simulink model "jacobian"  (R2024b)
settings: Solver=ode1  StartTime=0.0  StopTime=inf  FixedStep=dt  MaxStep=1/30  RelTol=1e-3
undefined symbols (not defined in the file or in its folder): alpha, f, J_inv, y0
libraries: instrumentlib x2, simulink x1
settings Model: Creator=root  LastModifiedBy=aalessan

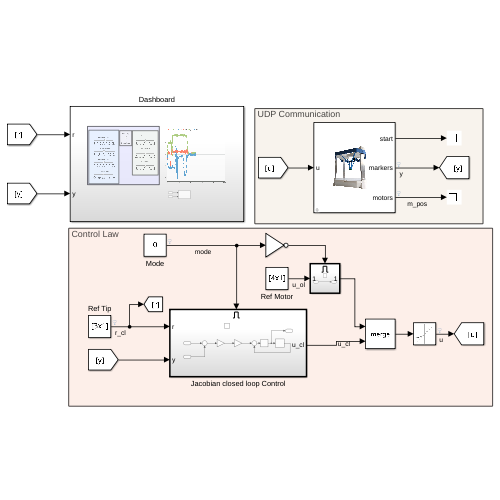
[thumbnail: Simulink's stored preview of the top-level diagram]
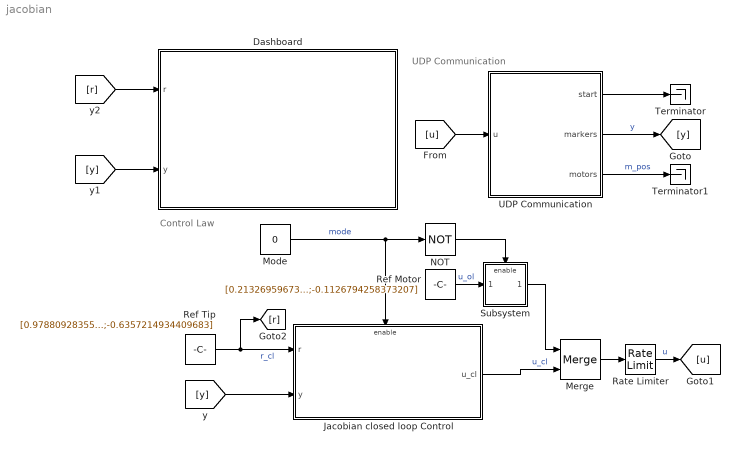
== system jacobian ==
  note: Control Law
  note: UDP Communication
  Dashboard : Subsystem
  Jacobian closed loop Control : Subsystem
  Merge : Merge  InitialOutput=zeros(4,1)
  Mode : Constant  Value=0
  NOT : Logic  Operator=NOT  IconShape=distinctive  AllPortsSameDT=off  OutDataTypeStr=boolean
  Rate Limiter : RateLimiter  RisingSlewLimit=7.906  FallingSlewLimit=-7.906  SampleTimeMode=inherited
  Ref Motor : Constant  Value=[0.213269596737653;-0.0957361805523107;-0.041409661167638;-0.1126794258373207]
  Ref Tip : Constant  Value=[0.9788092835519606;1.947527749747735;-0.6357214934409683]
  Subsystem : Subsystem
  Terminator : Terminator
  Terminator1 : Terminator
  UDP Communication : Subsystem  mask{nb_markers=1, markers_init=y0}
      mask prompts: nb_markers "Nb Markers"; markers_init "Initial Markers Position"
      mask Display: image('emio.png', [0,0,10,0,50,50]);
  wires:
  Merge/1 -> Rate Limiter/1
  Jacobian closed loop Control/1(u_cl) -> Merge/2  "u_cl"
  [u] -> UDP Communication/1(u)
  [y] -> Jacobian closed loop Control/2(y)
  Ref Tip/1 -> [r], Jacobian closed loop Control/1(r)  "r_cl"
  NOT/1 -> Subsystem/Enable
  Ref Motor/1 -> Subsystem/1(In1)  "u_ol"
  Mode/1 -> NOT/1, Jacobian closed loop Control/Enable  "mode"
  Subsystem/1(Out1) -> Merge/1
  Rate Limiter/1 -> [u]  "u"
  UDP Communication/3(motors) -> Terminator1/1  "m_pos"
  UDP Communication/1(start) -> Terminator/1
  UDP Communication/2(markers) -> [y]  "y"
  [y] -> Dashboard/2(y)
  [r] -> Dashboard/1(r)

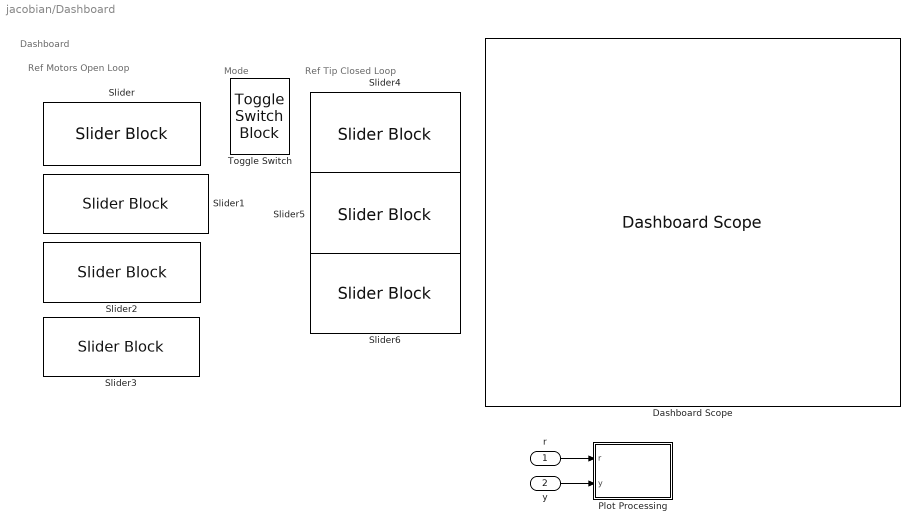
== system jacobian/Dashboard ==
  note: Mode
  note: Dashboard
  note: Ref Tip Closed Loop
  note: Ref Motors Open Loop
  r : Inport
  y : Inport  Port=2
  Dashboard Scope : DashboardScope  Ymin=-50  Ymax=50  UpdateMode=Scroll
  Plot Processing : Subsystem
  Slider{,1..3} (4 alike) : SliderBlock  ScaleMin=-1.57  ScaleMax=1.57
  Slider4 : SliderBlock  ScaleMin=-50  ScaleMax=50
  Slider5 : SliderBlock  ScaleMin=-50  ScaleMax=50
  Slider6 : SliderBlock  ScaleMin=-50  ScaleMax=50
  Toggle Switch : ToggleSwitchBlock  LabelPosition=Hide
      settings: Values={{'Closed Loop', 'Open Loop'}, [1 0]}
  wires:
  r/1 -> Plot Processing/1(r)
  y/1 -> Plot Processing/2(y)

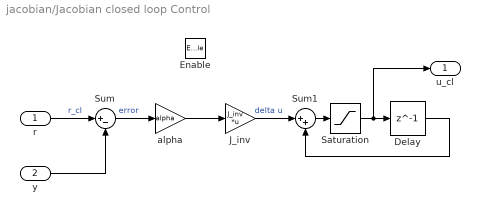
== system jacobian/Jacobian closed loop Control ==
  r : Inport
  y : Inport  Port=2
  Enable : EnablePort  StatesWhenEnabling=reset
  Delay : Delay  DelayLength=1  InitialCondition=zeros(4,1)
  J_inv : Gain  Gain=J_inv  Multiplication=Matrix(K*u)
  Saturation : Saturate  UpperLimit=1.57  LowerLimit=-1.57
  Sum : Sum  Inputs=|+-
  Sum1 : Sum  Inputs=|++
  alpha : Gain  Gain=alpha
  u_cl : Outport
  wires:
  Sum/1 -> alpha/1  "error"
  alpha/1 -> J_inv/1
  y/1 -> Sum/2
  r/1 -> Sum/1  "r_cl"
  J_inv/1 -> Sum1/1  "delta u"
  Delay/1 -> Sum1/2
  Sum1/1 -> Saturation/1
  Saturation/1 -> u_cl/1, Delay/1

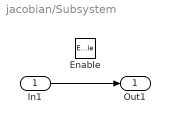
== system jacobian/Subsystem ==
  In1 : Inport
  Enable : EnablePort
  Out1 : Outport
  wires:
  In1/1 -> Out1/1

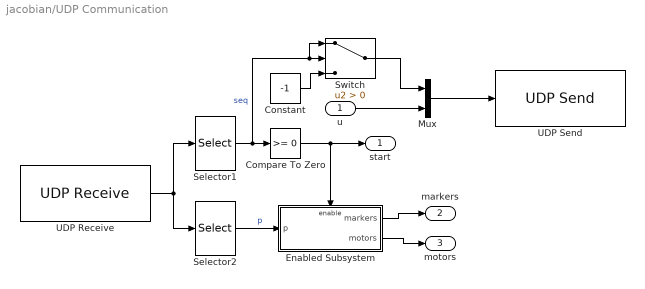
== system jacobian/UDP Communication ==
  u : Inport
  Compare To Zero : simulink/Logic and Bit Operations/Compare To Zero  relop=>=  OutDataTypeStr=boolean
  Constant : Constant  Value=-1
  Enabled Subsystem : Subsystem  TreatAsAtomicUnit=on
  Mux : Mux  Inputs=2
  Selector1 : Selector  InputPortWidth=5+3*nb_markers  IndexOptions=Index vector (dialog)  Indices=[1]  OutputSizes=1
  Selector2 : Selector  InputPortWidth=5+3*nb_markers  IndexOptions=Index vector (dialog)  Indices=2:5+3*nb_markers  OutputSizes=1
  Switch : Switch  Criteria=u2 > Threshold  SaturateOnIntegerOverflow=off  InputSameDT=off
  UDP Receive : instrumentlib/UDP Receive  LocalAddress=127.0.0.1  LocalPort=25000  EnablePortSharing=off  Host=127.0.0.1  Port=9090  GetLatestData=on  DataSize=[ 3*nb_markers+5, 1 ]  DataType=double  ASCIIFormatting=%f,  Terminator=LF  CustomTerminator=10  ByteOrder=little-endian  EnableBlockingMode=on  Timeout=0.1  SampleTime=-1  SimulateUsing=Interpreted execution
  UDP Send : instrumentlib/UDP Send  Host=127.0.0.1  Port=25001  LocalAddress=0.0.0.0  LocalPort=-1  EnablePortSharing=off  OutputDatagramPacketSize=512  ByteOrder=little-endian  EnableBlockingMode=on  SimulateUsing=Interpreted execution
  start : Outport
  markers : Outport  Port=2
  motors : Outport  Port=3
  wires:
  Mux/1 -> UDP Send/1
  u/1 -> Mux/2
  Enabled Subsystem/2(motors) -> motors/1
  Selector2/1 -> Enabled Subsystem/1(p)  "p"
  Enabled Subsystem/1(markers) -> markers/1
  Selector1/1 -> Switch/1, Switch/2, Compare To Zero/1  "seq"
  Compare To Zero/1 -> start/1, Enabled Subsystem/Enable
  Constant/1 -> Switch/3
  UDP Receive/1 -> Selector1/1, Selector2/1
  Switch/1 -> Mux/1

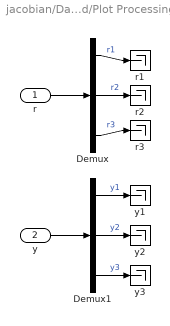
== system jacobian/Dashboard/Plot Processing ==
  r : Inport
  y : Inport  Port=2
  Demux : Demux  Outputs=3
  Demux1 : Demux  Outputs=3
  r1 : Terminator
  r2 : Terminator
  r3 : Terminator
  y1 : Terminator
  y2 : Terminator
  y3 : Terminator
  wires:
  Demux/1 -> r1/1  "r1"
  r/1 -> Demux/1
  Demux/2 -> r2/1  "r2"
  Demux/3 -> r3/1  "r3"
  y/1 -> Demux1/1
  Demux1/1 -> y1/1  "y1"
  Demux1/2 -> y2/1  "y2"
  Demux1/3 -> y3/1  "y3"

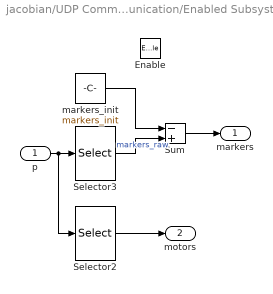
== system jacobian/UDP Communication/Enabled Subsystem ==
  p : Inport
  Enable : EnablePort
  Selector2 : Selector  InputPortWidth=4+3*nb_markers  IndexOptions=Index vector (dialog)  Indices=3*nb_markers+1:4+3*nb_markers  OutputSizes=1
  Selector3 : Selector  InputPortWidth=4+3*nb_markers  IndexOptions=Index vector (dialog)  Indices=1:3*nb_markers  OutputSizes=1
  Sum : Sum  Inputs=-+
  markers_init : Constant  Value=markers_init
  markers : Outport
  motors : Outport  Port=2
  wires:
  Sum/1 -> markers/1
  p/1 -> Selector2/1, Selector3/1
  Selector2/1 -> motors/1
  markers_init/1 -> Sum/1
  Selector3/1 -> Sum/2  "markers_raw"
